simulink model "sprint5"  (R2025b)
settings: Solver=VariableStepAuto  StartTime=0.0  StopTime=inf  RelTol=1e-3
undefined symbols (not defined in the file): gray
settings Model: Creator=juand  LastModifiedBy=valeriapinorivera

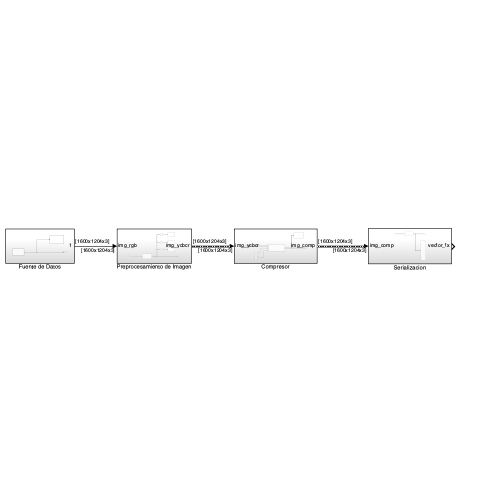
[thumbnail: Simulink's stored preview of the top-level diagram]
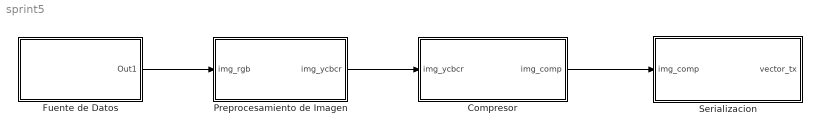
== system sprint5 ==
  Compresor : Subsystem
  Fuente de Datos : Subsystem
  Preprocesamiento de Imagen : Subsystem
  Serializacion : Subsystem
  wires:
  Fuente de Datos/1(Out1) -> Preprocesamiento de Imagen/1(img_rgb)
  Preprocesamiento de Imagen/1(img_ycbcr) -> Compresor/1(img_ycbcr)
  Compresor/1(img_comp) -> Serializacion/1(img_comp)

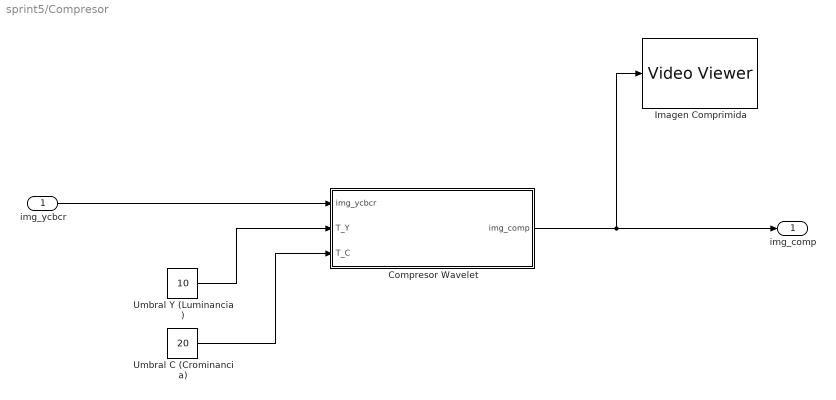
== system sprint5/Compresor ==
  img_ycbcr : Inport
  Compresor Wavelet : MATLAB Function  TreatAsAtomicUnit=on
  Imagen Comprimida : VideoViewer  colormapValue=gray(256)  FigPos=[1 910 1536 813]  OpenAtMdlStart=off
  Umbral C (Crominancia) : Constant  Value=20
  Umbral Y (Luminancia) : Constant  Value=10
  img_comp : Outport
  wires:
  Compresor Wavelet/1(img_comp) -> Imagen Comprimida/1, img_comp/1
  Umbral C (Crominancia)/1 -> Compresor Wavelet/3(T_C)
  Umbral Y (Luminancia)/1 -> Compresor Wavelet/2(T_Y)
  img_ycbcr/1 -> Compresor Wavelet/1(img_ycbcr)

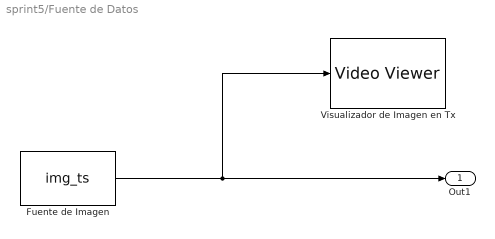
== system sprint5/Fuente de Datos ==
  Fuente de Imagen : FromWorkspace  VariableName=img_ts  SampleTime=1  Interpolate=off  ZeroCross=off  OutputAfterFinalValue=Holding final value
  Visualizador de Imagen en Tx : VideoViewer  FigPos=[559 631 418 304]  OpenAtMdlStart=off
  Out1 : Outport
  wires:
  Fuente de Imagen/1 -> Out1/1, Visualizador de Imagen en Tx/1

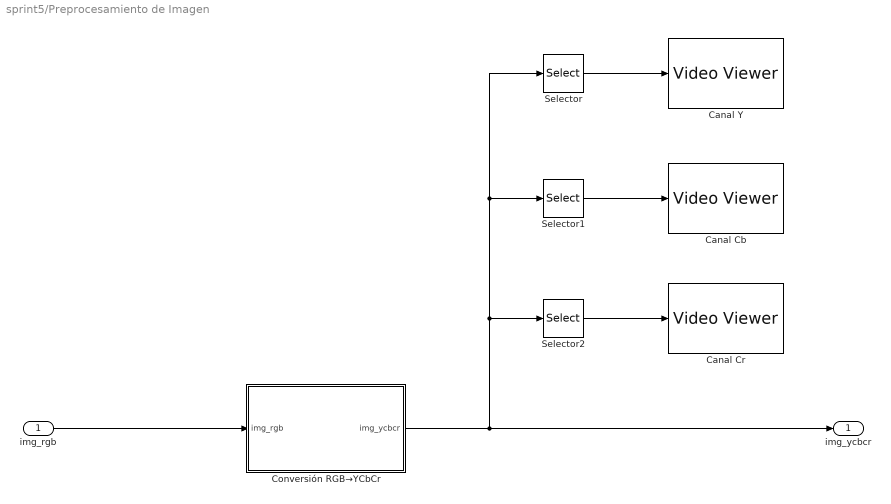
== system sprint5/Preprocesamiento de Imagen ==
  img_rgb : Inport
  Canal Cb : VideoViewer  colormapValue=gray(256)  FigPos=[559 631 418 304]  OpenAtMdlStart=off
  Canal Cr : VideoViewer  colormapValue=gray(256)  FigPos=[559 631 418 304]  OpenAtMdlStart=off
  Canal Y : VideoViewer  colormapValue=gray(256)  FigPos=[1 910 1536 813]  OpenAtMdlStart=off
  Conversión RGB→YCbCr : MATLAB Function  TreatAsAtomicUnit=on
  Selector : Selector  NumberOfDimensions=3  InputPortWidth=3  IndexOptions=Select all,Select all,Index vector (dialog)  Indices=[1 3],1,1  OutputSizes=1,1,1
  Selector1 : Selector  NumberOfDimensions=3  InputPortWidth=3  IndexOptions=Select all,Select all,Index vector (dialog)  Indices=[1 3],1,2  OutputSizes=1,1,1
  Selector2 : Selector  NumberOfDimensions=3  InputPortWidth=3  IndexOptions=Select all,Select all,Index vector (dialog)  Indices=[1 3],1,3  OutputSizes=1,1,1
  img_ycbcr : Outport
  wires:
  Conversión RGB→YCbCr/1(img_ycbcr) -> img_ycbcr/1, Selector2/1, Selector/1, Selector1/1
  Selector2/1 -> Canal Cr/1
  Selector/1 -> Canal Y/1
  Selector1/1 -> Canal Cb/1
  img_rgb/1 -> Conversión RGB→YCbCr/1(img_rgb)

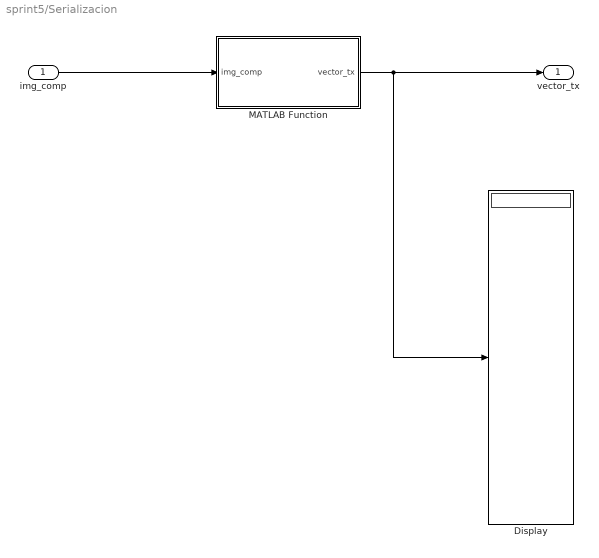
== system sprint5/Serializacion ==
  img_comp : Inport
  Display : Display
  MATLAB Function : MATLAB Function  TreatAsAtomicUnit=on
  vector_tx : Outport
  wires:
  img_comp/1 -> MATLAB Function/1(img_comp)
  MATLAB Function/1(vector_tx) -> Display/1, vector_tx/1

== matlab function sprint5/Compresor/Compresor Wavelet ==
  data: img_ycbcr input uint8 size=[1600 1204 3]; img_comp output double size=[1600 1204 3]; T_Y input double size=1; T_C input double size=1
function img_comp = bloque_wavelet_tx(img_ycbcr, T_Y, T_C)
%#codegen
% BLOQUE WAVELET Tx - Transformada Haar + Umbralización (3 canales)
%
% ENTRADAS:
%   img_ycbcr : imagen YCbCr, uint8, H x W x 3
%   T_Y       : umbral canal Y  (recomendado: 10)
%   T_C       : umbral Cb y Cr  (recomendado: 20)
%
% SALIDA:
%   img_comp  : imagen comprimida, double, H x W x 3

    [m, n, ~] = size(img_ycbcr);
    m2 = floor(m/2)*2;
    n2 = floor(n/2)*2;

    img_comp = zeros(m2, n2, 3);
    T = [T_Y, T_C, T_C];

    for c = 1:3
        I = double(img_ycbcr(1:m2, 1:n2, c));

        % Haar horizontal
        L = (I(:, 1:2:n2) + I(:, 2:2:n2)) / 2;
        H = (I(:, 1:2:n2) - I(:, 2:2:n2)) / 2;

        % Haar vertical
        LL = (L(1:2:m2,:) + L(2:2:m2,:)) / 2;
        LH = (L(1:2:m2,:) - L(2:2:m2,:)) / 2;
        HL = (H(1:2:m2,:) + H(2:2:m2,:)) / 2;
        HH = (H(1:2:m2,:) - H(2:2:m2,:)) / 2;

        % Umbralización
        LH(abs(LH) < T(c)) = 0;
        HL(abs(HL) < T(c)) = 0;
        HH(abs(HH) < T(c)) = 0;

        img_comp(:,:,c) = [LL, HL; LH, HH];
    end
end

== matlab function sprint5/Serializacion/MATLAB Function ==
  data: img_comp input double size=[1600 1204 3]; vector_tx output double size=[5779200 1]
function vector_tx = bloque_serializacion(img_comp)
%#codegen
% BLOQUE SERIALIZACIÓN - Imagen 3D → Vector 1D
% Va dentro del MATLAB Function block en Simulink.
%
% ENTRADA:
%   img_comp  : imagen comprimida, double, H x W x 3
%
% SALIDA:
%   vector_tx : vector serializado, double, (H*W*3) x 1

    vector_tx = img_comp(:);
end

== matlab function sprint5/Preprocesamiento de Imagen/Conversión RGB→YCbCr ==
  data: img_rgb input size=[1600 1204 3]; img_ycbcr output size=[1600 1204 3]
function img_ycbcr = bloque2_rgb_a_ycbcr(img_rgb)
%#codegen
% BLOQUE 2 - PREPROCESAMIENTO (Tx): RGB → YCbCr
% Va dentro del MATLAB Function block en Simulink.
%
% ENTRADA:
%   img_rgb   : imagen RGB,   uint8, H x W x 3
%
% SALIDA:
%   img_ycbcr : imagen YCbCr, uint8, H x W x 3
%               (:,:,1) = Y   luminancia
%               (:,:,2) = Cb  diferencia azul  (centro=128)
%               (:,:,3) = Cr  diferencia rojo  (centro=128)

    % --- Extraer canales R, G, B como double ---
    R = double(img_rgb(:,:,1));
    G = double(img_rgb(:,:,2));
    B = double(img_rgb(:,:,3));

    % --- Transformación RGB → YCbCr (ITU-R BT.601, full range) ---
    %
    % [ Y  ]   [ 0.2989   0.5870   0.1140 ] [ R ]   [   0 ]
    % [ Cb ] = [-0.1687  -0.3313   0.5000 ] [ G ] + [ 128 ]
    % [ Cr ]   [ 0.5000  -0.4187  -0.0813 ] [ B ]   [ 128 ]
    %
    Y_d  =  0.2989 * R + 0.5870 * G + 0.1140 * B;
    Cb_d = -0.1687 * R - 0.3313 * G + 0.5000 * B + 128.0;
    Cr_d =  0.5000 * R - 0.4187 * G - 0.0813 * B + 128.0;

    % --- Clip + conversión a uint8 ---
    Y  = uint8(max(0, min(255, Y_d)));
    Cb = uint8(max(0, min(255, Cb_d)));
    Cr = uint8(max(0, min(255, Cr_d)));

    % --- Apilar en un solo stack H x W x 3 ---
    img_ycbcr = cat(3, Y, Cb, Cr);
end
